simulink model "gm_kalman_ac_sim"  (R2025b)
settings: Solver=VariableStepAuto  StartTime=0.0  StopTime=StopTime  RelTol=1e-3
undefined symbols (not defined in the file or in its folder): dt, time
libraries: hdlmdlgenlib x45, hdlsllib x5, dspsrcs4 x3
settings Model: Creator=stefa  LastModifiedBy=david
settings OptimizationCC: BlockReduction=off  ConditionallyExecuteInputs=off
settings DebuggingCC: InheritedTsInSrcMsg=none

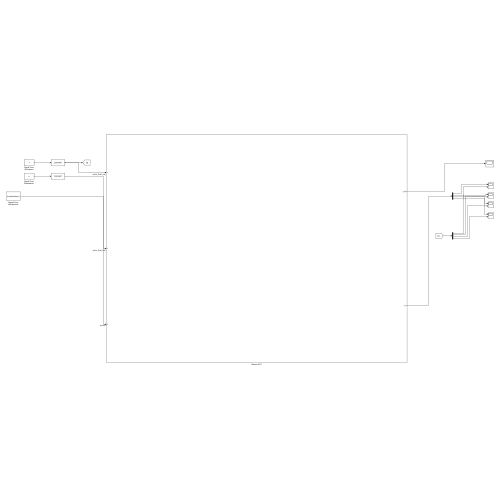
[thumbnail: Simulink's stored preview of the top-level diagram]
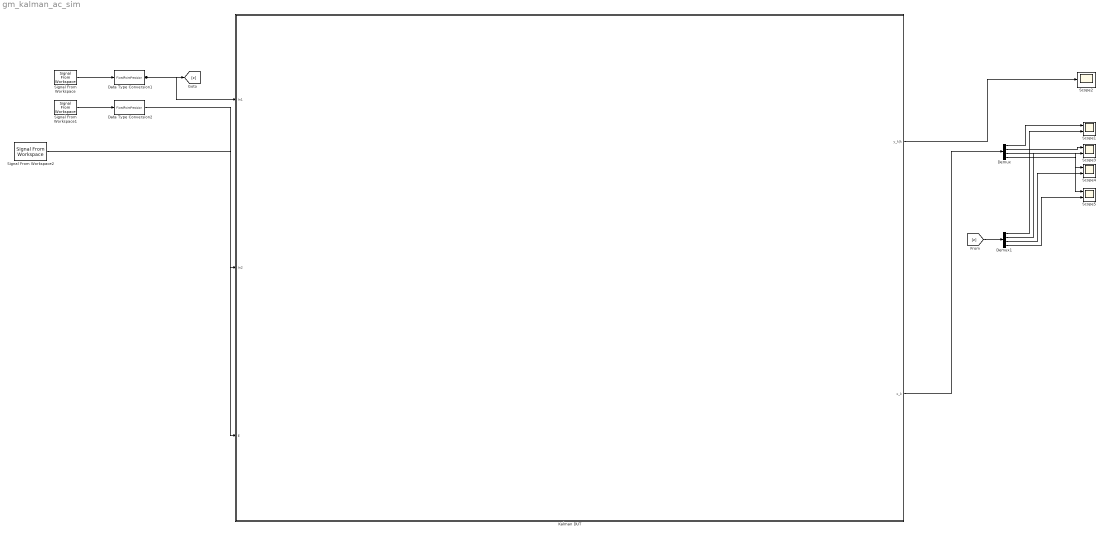
== system gm_kalman_ac_sim ==
  Data Type Conversion1 : DataTypeConversion  OutDataTypeStr=FixedPointPrecision  SaturateOnIntegerOverflow=off  RndMeth=Floor
  Data Type Conversion2 : DataTypeConversion  OutDataTypeStr=FixedPointPrecision  SaturateOnIntegerOverflow=off  RndMeth=Floor
  Demux : Demux
  Demux1 : Demux
  Kalman DUT : Subsystem
  Scope{1,3..5} (4 alike) : Scope  NumInputPorts=2
      Scope1 settings: ActiveDisplayYMinimum=0.44600438166261591  ActiveDisplayYMaximum=2.0535397271105578  DataLoggingSaveFormat=Array
      Scope3 settings: ActiveDisplayYMinimum=-1  ActiveDisplayYMaximum=1  DataLoggingVariableName=ScopeData2  DataLoggingSaveFormat=Array
      Scope4 settings: ActiveDisplayYMinimum=-2.08087494415443  ActiveDisplayYMaximum=12.219950065546442  DataLoggingVariableName=ScopeData3  DataLoggingSaveFormat=Array
      Scope5 settings: ActiveDisplayYMinimum=-0.36244737237361535  ActiveDisplayYMaximum=0.44371345235011872  DataLoggingVariableName=ScopeData4  DataLoggingSaveFormat=Array
  Scope2 : Scope
      settings: ActiveDisplayYMinimum=-0.011525178669385456  ActiveDisplayYMaximum=0.00587966952456793  DataLoggingSaveFormat=Array
  Signal From Workspace : dspsrcs4/Signal From Workspace  X=z  Ts=dt  nsamps=1  OutputAfterFinalValue=Setting to zero  ignoreOrWarnInputAndFrameLengths=off  OutputFrames=off
  Signal From Workspace1 : dspsrcs4/Signal From Workspace  X=u  Ts=dt  nsamps=1  OutputAfterFinalValue=Setting to zero  ignoreOrWarnInputAndFrameLengths=off  OutputFrames=off
  Signal From Workspace2 : dspsrcs4/Signal From Workspace  X=true(size(time))  Ts=dt  nsamps=1  OutputAfterFinalValue=Setting to zero  ignoreOrWarnInputAndFrameLengths=off  OutputFrames=off
  wires:
  Signal From Workspace2/1 -> Kalman DUT/3(E)
  Data Type Conversion2/1 -> Kalman DUT/2(In2)
  Data Type Conversion1/1 -> [z], Kalman DUT/1(In1)
  Kalman DUT/2(x_k) -> Demux/1
  Kalman DUT/1(y_k|k) -> Scope2/1
  Signal From Workspace1/1 -> Data Type Conversion2/1
  Signal From Workspace/1 -> Data Type Conversion1/1
  Demux1/4 -> Scope5/2
  Demux1/3 -> Scope4/2
  Demux1/2 -> Scope3/2
  Demux1/1 -> Scope1/2
  [z] -> Demux1/1
  Demux/4 -> Scope5/1
  Demux/3 -> Scope4/1
  Demux/2 -> Scope3/1
  Demux/1 -> Scope1/1

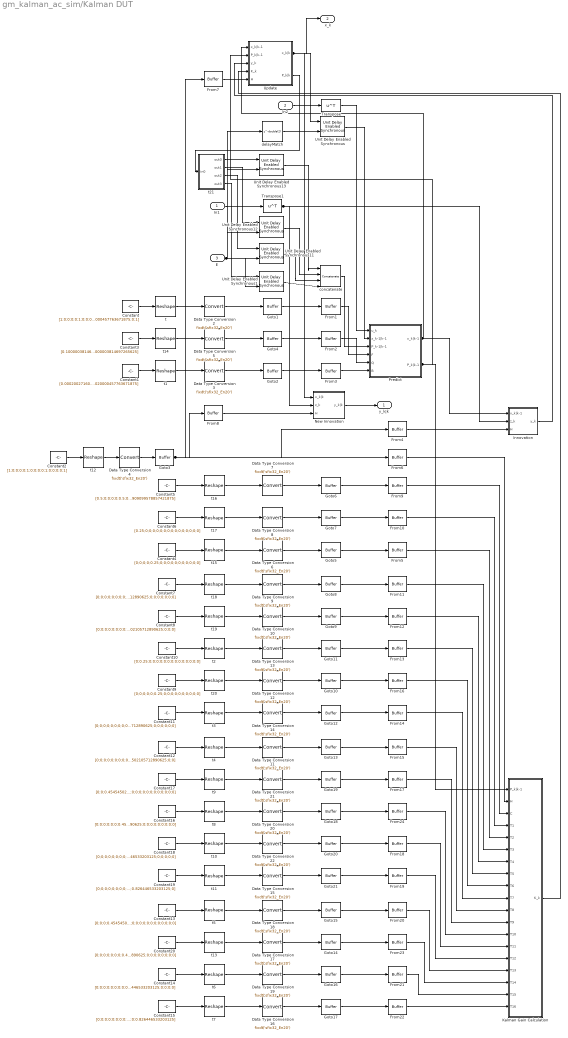
== system gm_kalman_ac_sim/Kalman DUT ==
  In1 : Inport  OutDataTypeStr=fixdt(1, 32, 20)  PortDimensions=[1 4]  SampleTime=0.02
  In2 : Inport  Port=2  OutDataTypeStr=fixdt(1, 32, 20)  PortDimensions=[1 2]  SampleTime=0.02
  E : Inport  Port=3  OutDataTypeStr=boolean  PortDimensions=1  SampleTime=0.02
  Constant : Constant  Value=[1;0;0;0;0;1;0;0;0.020000457763671875;0;1;0;0;0.020000457763671875;0;1]  OutDataTypeStr=fixdt(1, 32, 20)  SampleTime=0.02
  Constant1 : Constant  Value=[0.0002002716064453125;0;0.020000457763671875;0;0;0.0002002716064453125;0;0.020000457763671875]  OutDataTypeStr=fixdt(1, 32, 20)  SampleTime=0.02
  Constant10 : Constant  Value=[0;0.25;0;0;0;0;0;0;0;0;0;0;0;0;0;0]  OutDataTypeStr=fixdt(1, 32, 20)  SampleTime=0.02
  Constant11 : Constant  Value=[0;0;0;0;0;0;0;0;0;0.45454502105712890625;0;0;0;0;0;0]  OutDataTypeStr=fixdt(1, 32, 20)  SampleTime=0.02
  Constant12 : Constant  Value=[0;0;0;0;0;0;0;0;0;0;0;0;0;0.45454502105712890625;0;0]  OutDataTypeStr=fixdt(1, 32, 20)  SampleTime=0.02
  Constant13 : Constant  Value=[0;0;0;0.45454502105712890625;0;0;0;0;0;0;0;0;0;0;0;0]  OutDataTypeStr=fixdt(1, 32, 20)  SampleTime=0.02
  Constant14 : Constant  Value=[0;0;0;0;0;0;0;0;0;0;0;0.826446533203125;0;0;0;0]  OutDataTypeStr=fixdt(1, 32, 20)  SampleTime=0.02
  Constant15 : Constant  Value=[0;0;0;0;0;0;0;0;0;0;0;0;0;0;0;0.826446533203125]  OutDataTypeStr=fixdt(1, 32, 20)  SampleTime=0.02
  Constant16 : Constant  Value=[0;0;0;0;0;0;0.45454502105712890625;0;0;0;0;0;0;0;0;0]  OutDataTypeStr=fixdt(1, 32, 20)  SampleTime=0.02
  Constant17 : Constant  Value=[0;0;0.45454502105712890625;0;0;0;0;0;0;0;0;0;0;0;0;0]  OutDataTypeStr=fixdt(1, 32, 20)  SampleTime=0.02
  Constant18 : Constant  Value=[0;0;0;0;0;0;0;0;0;0;0.826446533203125;0;0;0;0;0]  OutDataTypeStr=fixdt(1, 32, 20)  SampleTime=0.02
  Constant19 : Constant  Value=[0;0;0;0;0;0;0;0;0;0;0;0;0;0;0.826446533203125;0]  OutDataTypeStr=fixdt(1, 32, 20)  SampleTime=0.02
  Constant2 : Constant  Value=[1;0;0;0;0;1;0;0;0;0;1;0;0;0;0;1]  OutDataTypeStr=fixdt(1, 32, 20)  SampleTime=0.02
  Constant20 : Constant  Value=[0;0;0;0;0;0;0;0.45454502105712890625;0;0;0;0;0;0;0;0]  OutDataTypeStr=fixdt(1, 32, 20)  SampleTime=0.02
  Constant3 : Constant  Value=[0.1000003814697265625;0;0;0;0;0.1000003814697265625;0;0;0;0;0.1000003814697265625;0;0;0;0;0.1000003814697265625]  OutDataTypeStr=fixdt(1, 32, 20)  SampleTime=0.02
  Constant4 : Constant  Value=[0;0;0;0;0.25;0;0;0;0;0;0;0;0;0;0;0]  OutDataTypeStr=fixdt(1, 32, 20)  SampleTime=0.02
  Constant5 : Constant  Value=[0.5;0;0;0;0;0.5;0;0;0;0;0.90909099578857421875;0;0;0;0;0.90909099578857421875]  OutDataTypeStr=fixdt(1, 32, 20)  SampleTime=0.02
  Constant6 : Constant  Value=[0.25;0;0;0;0;0;0;0;0;0;0;0;0;0;0;0]  OutDataTypeStr=fixdt(1, 32, 20)  SampleTime=0.02
  Constant7 : Constant  Value=[0;0;0;0;0;0;0;0;0.45454502105712890625;0;0;0;0;0;0;0]  OutDataTypeStr=fixdt(1, 32, 20)  SampleTime=0.02
  Constant8 : Constant  Value=[0;0;0;0;0;0;0;0;0;0;0;0;0.45454502105712890625;0;0;0]  OutDataTypeStr=fixdt(1, 32, 20)  SampleTime=0.02
  Constant9 : Constant  Value=[0;0;0;0;0;0.25;0;0;0;0;0;0;0;0;0;0]  OutDataTypeStr=fixdt(1, 32, 20)  SampleTime=0.02
  Data Type Conversion{2..22} (21 alike) : DataTypeConversion  OutDataTypeStr=fixdt('sfix32_En20')
  From{1..24} (24 alike) : hdlmdlgenlib/Buffer
  Goto{1..21} (21 alike) : hdlmdlgenlib/Buffer
  Innovation : Subsystem
  Kalman Gain Calculation : Subsystem
  New Innovation : Subsystem
  Predict : Subsystem
  Transpose : Math  Operator=transpose  SignedPower=on  OutDataTypeStr=fixdt(1, 32, 20)  RndMeth=Zero
  Transpose1 : Math  Operator=transpose  SignedPower=on  OutDataTypeStr=fixdt(1, 32, 20)  RndMeth=Zero
  Unit Delay Enabled Synchronous{,1,11..13} (5 alike) : hdlsllib/Discrete/Unit Delay Enabled Synchronous  InitialCondition=double(0)  SampleTime=-1
  Update : Subsystem
  concatenate : Concatenate  NumInputs=4  Mode=Multidimensional array  ConcatenateDimension=2
  delayMatch : Delay  DelayLength=double(2)  InitialCondition=0  SampleTime=0.02
  t{,2..20} (20 alike) : Reshape  OutputDimensionality=Customize  OutputDimensions=[4,4]
  t1 : Reshape  OutputDimensionality=Customize  OutputDimensions=[4,2]
  t21 : Subsystem
  y_k|k : Outport  SampleTime=0.02
  x_k : Outport  Port=2  SampleTime=0.02
  wires:
  t14/1 -> Data Type Conversion5/1
  From7/1 -> Update/5(H)
  Constant2/1 -> t12/1
  t21/2(out1) -> Unit Delay Enabled Synchronous12/1
  Constant1/1 -> t1/1
  t10/1 -> Data Type Conversion22/1
  Goto3/1 -> From6/1, From7/1, From8/1, From4/1
  t12/1 -> Data Type Conversion4/1
  Constant/1 -> t/1
  Constant5/1 -> t16/1
  t6/1 -> Data Type Conversion19/1
  Constant4/1 -> t15/1
  Constant6/1 -> t17/1
  Constant3/1 -> t14/1
  Data Type Conversion4/1 -> Goto3/1
  t/1 -> Data Type Conversion2/1
  delayMatch/1 -> Unit Delay Enabled Synchronous/2
  t1/1 -> Data Type Conversion3/1
  t4/1 -> Data Type Conversion11/1
  From18/1 -> Kalman Gain Calculation/14(T11)
  t2/1 -> Data Type Conversion13/1
  Constant9/1 -> t20/1
  Constant8/1 -> t19/1
  Constant7/1 -> t18/1
  Constant13/1 -> t5/1
  Constant12/1 -> t4/1
  Constant11/1 -> t3/1
  Constant10/1 -> t2/1
  Constant14/1 -> t6/1
  Constant17/1 -> t9/1
  Unit Delay Enabled Synchronous12/1 -> concatenate/2
  From16/1 -> Kalman Gain Calculation/9(T6)
  t9/1 -> Data Type Conversion21/1
  Constant20/1 -> t13/1
  Constant16/1 -> t8/1
  Constant19/1 -> t11/1
  Constant18/1 -> t10/1
  Transpose1/1 -> Innovation/2(z_k), New Innovation/2(z_k)
  Goto11/1 -> From13/1
  Constant15/1 -> t7/1
  t21/1(out0) -> Unit Delay Enabled Synchronous13/1
  t21/3(out2) -> Unit Delay Enabled Synchronous11/1
  t21/4(out3) -> Unit Delay Enabled Synchronous1/1
  In1/1 -> Transpose1/1
  E/1 -> delayMatch/1, Unit Delay Enabled Synchronous13/2, Unit Delay Enabled Synchronous11/2, Unit Delay Enabled Synchronous12/2, Unit Delay Enabled Synchronous1/2
  Data Type Conversion2/1 -> Goto1/1
  Data Type Conversion5/1 -> Goto4/1
  Data Type Conversion3/1 -> Goto2/1
  From8/1 -> New Innovation/3(H)
  t16/1 -> Data Type Conversion7/1
  t17/1 -> Data Type Conversion8/1
  t13/1 -> Data Type Conversion17/1
  t15/1 -> Data Type Conversion6/1
  Unit Delay Enabled Synchronous13/1 -> concatenate/1
  t20/1 -> Data Type Conversion12/1
  Goto8/1 -> From11/1
  t18/1 -> Data Type Conversion9/1
  t19/1 -> Data Type Conversion10/1
  t3/1 -> Data Type Conversion14/1
  t8/1 -> Data Type Conversion20/1
  t11/1 -> Data Type Conversion15/1
  Goto5/1 -> From5/1
  t7/1 -> Data Type Conversion16/1
  t5/1 -> Data Type Conversion18/1
  Update/1(x_k|k) -> Unit Delay Enabled Synchronous/1, New Innovation/1(x_k|k), x_k/1
  Update/2(P_k|k) -> t21/1(in0)
  Unit Delay Enabled Synchronous1/1 -> concatenate/4
  In2/1 -> Transpose/1
  Unit Delay Enabled Synchronous11/1 -> concatenate/3
  Predict/2(P_k|k-1) -> Update/2(P_k|k-1), Kalman Gain Calculation/1(P_k|k-1)
  Goto1/1 -> From1/1
  Goto4/1 -> From2/1
  Goto2/1 -> From3/1
  Data Type Conversion7/1 -> Goto6/1
  Data Type Conversion8/1 -> Goto7/1
  Data Type Conversion6/1 -> Goto5/1
  Data Type Conversion9/1 -> Goto8/1
  Data Type Conversion10/1 -> Goto9/1
  Data Type Conversion13/1 -> Goto11/1
  Data Type Conversion12/1 -> Goto10/1
  Data Type Conversion14/1 -> Goto12/1
  Data Type Conversion11/1 -> Goto13/1
  Data Type Conversion21/1 -> Goto19/1
  Data Type Conversion20/1 -> Goto18/1
  Data Type Conversion22/1 -> Goto20/1
  From23/1 -> Kalman Gain Calculation/17(T14)
  Unit Delay Enabled Synchronous/1 -> Predict/2(x_k-1|k-1)
  Data Type Conversion15/1 -> Goto21/1
  Data Type Conversion18/1 -> Goto15/1
  Data Type Conversion17/1 -> Goto14/1
  Data Type Conversion19/1 -> Goto16/1
  Data Type Conversion16/1 -> Goto17/1
  Transpose/1 -> Predict/1(u_k)
  concatenate/1 -> Predict/3(P_k-1|k-1)
  From1/1 -> Predict/4(F)
  From2/1 -> Predict/5(Q)
  From3/1 -> Predict/6(B)
  New Innovation/1(y_k|k) -> y_k|k/1
  Goto6/1 -> From9/1
  Goto7/1 -> From10/1
  Goto9/1 -> From12/1
  Goto10/1 -> From16/1
  Goto12/1 -> From14/1
  Goto13/1 -> From15/1
  Goto19/1 -> From17/1
  Goto18/1 -> From24/1
  Goto20/1 -> From18/1
  Goto21/1 -> From19/1
  Goto15/1 -> From20/1
  Goto14/1 -> From23/1
  Goto16/1 -> From21/1
  Goto17/1 -> From22/1
  Predict/1(x_k|k-1) -> Update/1(x_k|k-1), Innovation/1(x_k|k-1)
  From4/1 -> Innovation/3(H)
  From6/1 -> Kalman Gain Calculation/2(H)
  From9/1 -> Kalman Gain Calculation/3(C)
  From10/1 -> Kalman Gain Calculation/4(T1)
  From5/1 -> Kalman Gain Calculation/5(T2)
  From11/1 -> Kalman Gain Calculation/6(T3)
  From12/1 -> Kalman Gain Calculation/7(T4)
  From13/1 -> Kalman Gain Calculation/8(T5)
  From14/1 -> Kalman Gain Calculation/10(T7)
  From15/1 -> Kalman Gain Calculation/11(T8)
  From17/1 -> Kalman Gain Calculation/12(T9)
  From24/1 -> Kalman Gain Calculation/13(T10)
  From19/1 -> Kalman Gain Calculation/15(T12)
  From20/1 -> Kalman Gain Calculation/16(T13)
  From21/1 -> Kalman Gain Calculation/18(T15)
  From22/1 -> Kalman Gain Calculation/19(T16)
  Innovation/1(y_k) -> Update/3(y_k)
  Kalman Gain Calculation/1(K_k) -> Update/4(K_k)

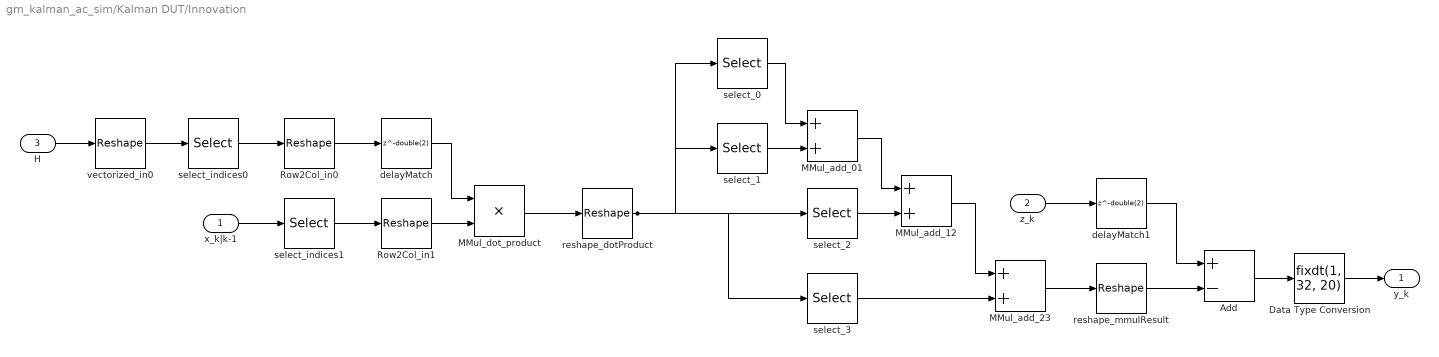
== system gm_kalman_ac_sim/Kalman DUT/Innovation ==
  x_k|k-1 : Inport  OutDataTypeStr=fixdt(1, 32, 20)  PortDimensions=[4 1]  SampleTime=0.02
  z_k : Inport  Port=2  OutDataTypeStr=fixdt(1, 32, 20)  PortDimensions=[4 1]  SampleTime=0.02
  H : Inport  Port=3  OutDataTypeStr=fixdt(1, 32, 20)  PortDimensions=[4,4]  SampleTime=0.02
  Add : Sum  Inputs=+-  OutDataTypeStr=fixdt(1, 64, 40)  AccumDataTypeStr=fixdt(1, 64, 40)  SampleTime=0.02
  Data Type Conversion : DataTypeConversion  OutDataTypeStr=fixdt(1, 32, 20)  SampleTime=0.02  SaturateOnIntegerOverflow=off  RndMeth=Floor
  MMul_add_01 : Sum  OutDataTypeStr=fixdt(1, 64, 40)  SampleTime=0.02
  MMul_add_12 : Sum  OutDataTypeStr=fixdt(1, 64, 40)  SampleTime=0.02
  MMul_add_23 : Sum  OutDataTypeStr=fixdt(1, 64, 40)  SampleTime=0.02
  MMul_dot_product : Product  Inputs=**  OutDataTypeStr=fixdt(1, 64, 40)  SampleTime=0.02
  Row2Col_in0 : Reshape  OutputDimensionality=Column vector (2-D)
  Row2Col_in1 : Reshape  OutputDimensionality=Column vector (2-D)
  delayMatch : Delay  DelayLength=double(2)  InitialCondition=0  SampleTime=0.02
  delayMatch1 : Delay  DelayLength=double(2)  InitialCondition=0  SampleTime=0.02
  reshape_dotProduct : Reshape  OutputDimensionality=Customize  OutputDimensions=[4,4]
  reshape_mmulResult : Reshape  OutputDimensionality=Customize  OutputDimensions=[4,1]
  select_0 : Selector  NumberOfDimensions=2  IndexOptions=Index vector (dialog),Select all  Indices=double(1),[]  OutputSizes=1
  select_1 : Selector  NumberOfDimensions=2  IndexOptions=Index vector (dialog),Select all  Indices=double(2),[]  OutputSizes=1
  select_2 : Selector  NumberOfDimensions=2  IndexOptions=Index vector (dialog),Select all  Indices=double(3),[]  OutputSizes=1
  select_3 : Selector  NumberOfDimensions=2  IndexOptions=Index vector (dialog),Select all  Indices=double(4),[]  OutputSizes=1
  select_indices0 : Selector  InputPortWidth=16  IndexOptions=Index vector (dialog)  Indices=double([1;5;9;13;2;6;10;14;3;7;11;15;4;8;12;16])  OutputSizes=1
  select_indices1 : Selector  InputPortWidth=4  IndexOptions=Index vector (dialog)  Indices=double([1;2;3;4;1;2;3;4;1;2;3;4;1;2;3;4])  OutputSizes=1
  vectorized_in0 : Reshape  OutputDimensionality=Row vector (2-D)
  y_k : Outport  SampleTime=0.02
  wires:
  H/1 -> vectorized_in0/1
  vectorized_in0/1 -> select_indices0/1
  select_indices0/1 -> Row2Col_in0/1
  Row2Col_in0/1 -> delayMatch/1
  MMul_add_23/1 -> reshape_mmulResult/1
  delayMatch/1 -> MMul_dot_product/1
  x_k|k-1/1 -> select_indices1/1
  Row2Col_in1/1 -> MMul_dot_product/2
  select_indices1/1 -> Row2Col_in1/1
  MMul_dot_product/1 -> reshape_dotProduct/1
  reshape_dotProduct/1 -> select_3/1, select_1/1, select_2/1, select_0/1
  select_0/1 -> MMul_add_01/1
  select_1/1 -> MMul_add_01/2
  MMul_add_01/1 -> MMul_add_12/1
  select_2/1 -> MMul_add_12/2
  select_3/1 -> MMul_add_23/2
  MMul_add_12/1 -> MMul_add_23/1
  z_k/1 -> delayMatch1/1
  delayMatch1/1 -> Add/1
  reshape_mmulResult/1 -> Add/2
  Add/1 -> Data Type Conversion/1
  Data Type Conversion/1 -> y_k/1

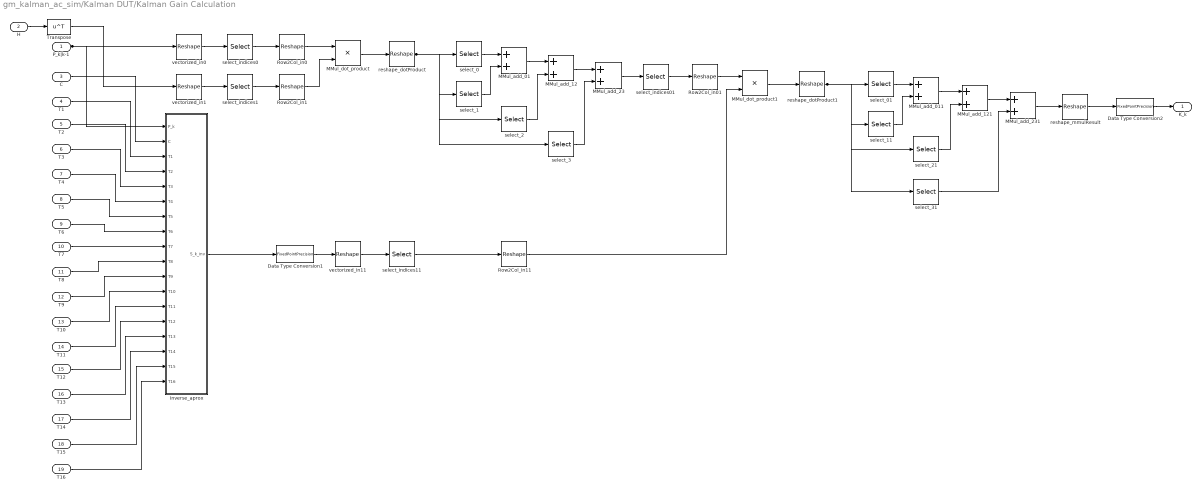
== system gm_kalman_ac_sim/Kalman DUT/Kalman Gain Calculation ==
  P_k|k-1 : Inport  OutDataTypeStr=fixdt(1, 32, 20)  PortDimensions=[4,4]  SampleTime=0.02
  H : Inport  Port=2  OutDataTypeStr=fixdt(1, 32, 20)  PortDimensions=[4,4]  SampleTime=0.02
  C : Inport  Port=3  OutDataTypeStr=fixdt(1, 32, 20)  PortDimensions=[4,4]  SampleTime=0.02
  T1 : Inport  Port=4  OutDataTypeStr=fixdt(1, 32, 20)  PortDimensions=[4,4]  SampleTime=0.02
  T2 : Inport  Port=5  OutDataTypeStr=fixdt(1, 32, 20)  PortDimensions=[4,4]  SampleTime=0.02
  T3 : Inport  Port=6  OutDataTypeStr=fixdt(1, 32, 20)  PortDimensions=[4,4]  SampleTime=0.02
  T4 : Inport  Port=7  OutDataTypeStr=fixdt(1, 32, 20)  PortDimensions=[4,4]  SampleTime=0.02
  T5 : Inport  Port=8  OutDataTypeStr=fixdt(1, 32, 20)  PortDimensions=[4,4]  SampleTime=0.02
  T6 : Inport  Port=9  OutDataTypeStr=fixdt(1, 32, 20)  PortDimensions=[4,4]  SampleTime=0.02
  T7 : Inport  Port=10  OutDataTypeStr=fixdt(1, 32, 20)  PortDimensions=[4,4]  SampleTime=0.02
  T8 : Inport  Port=11  OutDataTypeStr=fixdt(1, 32, 20)  PortDimensions=[4,4]  SampleTime=0.02
  T9 : Inport  Port=12  OutDataTypeStr=fixdt(1, 32, 20)  PortDimensions=[4,4]  SampleTime=0.02
  T10 : Inport  Port=13  OutDataTypeStr=fixdt(1, 32, 20)  PortDimensions=[4,4]  SampleTime=0.02
  T11 : Inport  Port=14  OutDataTypeStr=fixdt(1, 32, 20)  PortDimensions=[4,4]  SampleTime=0.02
  T12 : Inport  Port=15  OutDataTypeStr=fixdt(1, 32, 20)  PortDimensions=[4,4]  SampleTime=0.02
  T13 : Inport  Port=16  OutDataTypeStr=fixdt(1, 32, 20)  PortDimensions=[4,4]  SampleTime=0.02
  T14 : Inport  Port=17  OutDataTypeStr=fixdt(1, 32, 20)  PortDimensions=[4,4]  SampleTime=0.02
  T15 : Inport  Port=18  OutDataTypeStr=fixdt(1, 32, 20)  PortDimensions=[4,4]  SampleTime=0.02
  T16 : Inport  Port=19  OutDataTypeStr=fixdt(1, 32, 20)  PortDimensions=[4,4]  SampleTime=0.02
  Data Type Conversion1 : DataTypeConversion  OutDataTypeStr=FixedPointPrecision  SaturateOnIntegerOverflow=off  RndMeth=Floor
  Data Type Conversion2 : DataTypeConversion  OutDataTypeStr=FixedPointPrecision  SaturateOnIntegerOverflow=off  RndMeth=Floor
  Inverse_aprox : Subsystem
  MMul_add_01 : Sum  OutDataTypeStr=fixdt(1, 64, 40)  SampleTime=0.02
  MMul_add_011 : Sum  OutDataTypeStr=fixdt(1, 96, 60)  SampleTime=0.02
  MMul_add_12 : Sum  OutDataTypeStr=fixdt(1, 64, 40)  SampleTime=0.02
  MMul_add_121 : Sum  OutDataTypeStr=fixdt(1, 96, 60)  SampleTime=0.02
  MMul_add_23 : Sum  OutDataTypeStr=fixdt(1, 64, 40)  SampleTime=0.02
  MMul_add_231 : Sum  OutDataTypeStr=fixdt(1, 96, 60)  SampleTime=0.02
  MMul_dot_product : Product  Inputs=**  OutDataTypeStr=fixdt(1, 64, 40)  SampleTime=0.02
  MMul_dot_product1 : Product  Inputs=**  OutDataTypeStr=fixdt(1, 96, 60)  SampleTime=0.02
  Row2Col_in0 : Reshape  OutputDimensionality=Column vector (2-D)
  Row2Col_in01 : Reshape  OutputDimensionality=Column vector (2-D)
  Row2Col_in1 : Reshape  OutputDimensionality=Column vector (2-D)
  Row2Col_in11 : Reshape  OutputDimensionality=Column vector (2-D)
  Transpose : Math  Operator=transpose  SignedPower=on  OutDataTypeStr=fixdt(1, 32, 20)  RndMeth=Zero
  reshape_dotProduct : Reshape  OutputDimensionality=Customize  OutputDimensions=[4,16]
  reshape_dotProduct1 : Reshape  OutputDimensionality=Customize  OutputDimensions=[4,16]
  reshape_mmulResult : Reshape  OutputDimensionality=Customize  OutputDimensions=[4,4]
  select_0 : Selector  NumberOfDimensions=2  IndexOptions=Index vector (dialog),Select all  Indices=double(1),[]  OutputSizes=1
  select_01 : Selector  NumberOfDimensions=2  IndexOptions=Index vector (dialog),Select all  Indices=double(1),[]  OutputSizes=1
  select_1 : Selector  NumberOfDimensions=2  IndexOptions=Index vector (dialog),Select all  Indices=double(2),[]  OutputSizes=1
  select_11 : Selector  NumberOfDimensions=2  IndexOptions=Index vector (dialog),Select all  Indices=double(2),[]  OutputSizes=1
  select_2 : Selector  NumberOfDimensions=2  IndexOptions=Index vector (dialog),Select all  Indices=double(3),[]  OutputSizes=1
  select_21 : Selector  NumberOfDimensions=2  IndexOptions=Index vector (dialog),Select all  Indices=double(3),[]  OutputSizes=1
  select_3 : Selector  NumberOfDimensions=2  IndexOptions=Index vector (dialog),Select all  Indices=double(4),[]  OutputSizes=1
  select_31 : Selector  NumberOfDimensions=2  IndexOptions=Index vector (dialog),Select all  Indices=double(4),[]  OutputSizes=1
  select_indices0 : Selector  InputPortWidth=16  IndexOptions=Index vector (dialog)  Indices=double([1;5;9;13;2;6;10;14;3;7;11;15;4;8;12;16;1;5;9;13;2;6;10;14;3;7;11;15;4;8;12;16;1;5;9;13;2;6;10;14;3;7;11;15;4;8;12;16;1;5;9;13;2;6;10;14;3;7;11;15;4;8;12;16])  OutputSizes=1
  select_indices01 : Selector  InputPortWidth=16  IndexOptions=Index vector (dialog)  Indices=double([1;5;9;13;2;6;10;14;3;7;11;15;4;8;12;16;1;5;9;13;2;6;10;14;3;7;11;15;4;8;12;16;1;5;9;13;2;6;10;14;3;7;11;15;4;8;12;16;1;5;9;13;2;6;10;14;3;7;11;15;4;8;12;16])  OutputSizes=1
  select_indices1 : Selector  InputPortWidth=16  IndexOptions=Index vector (dialog)  Indices=double([1;2;3;4;1;2;3;4;1;2;3;4;1;2;3;4;5;6;7;8;5;6;7;8;5;6;7;8;5;6;7;8;9;10;11;12;9;10;11;12;9;10;11;12;9;10;11;12;13;14;15;16;13;14;15;16;13;14;15;16;13;14;15;16])  OutputSizes=1
  select_indices11 : Selector  InputPortWidth=16  IndexOptions=Index vector (dialog)  Indices=double([1;2;3;4;1;2;3;4;1;2;3;4;1;2;3;4;5;6;7;8;5;6;7;8;5;6;7;8;5;6;7;8;9;10;11;12;9;10;11;12;9;10;11;12;9;10;11;12;13;14;15;16;13;14;15;16;13;14;15;16;13;14;15;16])  OutputSizes=1
  vectorized_in0 : Reshape  OutputDimensionality=Row vector (2-D)
  vectorized_in1 : Reshape  OutputDimensionality=Row vector (2-D)
  vectorized_in11 : Reshape  OutputDimensionality=Row vector (2-D)
  K_k : Outport  SampleTime=0.02
  wires:
  C/1 -> Inverse_aprox/2(C)
  Row2Col_in1/1 -> MMul_dot_product/2
  H/1 -> Transpose/1
  Transpose/1 -> vectorized_in1/1
  P_k|k-1/1 -> Inverse_aprox/1(P_k), vectorized_in0/1
  MMul_dot_product/1 -> reshape_dotProduct/1
  T1/1 -> Inverse_aprox/3(T1)
  T3/1 -> Inverse_aprox/5(T3)
  reshape_dotProduct/1 -> select_3/1, select_2/1, select_0/1, select_1/1
  T2/1 -> Inverse_aprox/4(T2)
  select_1/1 -> MMul_add_01/2
  T6/1 -> Inverse_aprox/8(T6)
  T4/1 -> Inverse_aprox/6(T4)
  select_0/1 -> MMul_add_01/1
  T5/1 -> Inverse_aprox/7(T5)
  MMul_add_12/1 -> MMul_add_23/1
  select_2/1 -> MMul_add_12/2
  T7/1 -> Inverse_aprox/9(T7)
  MMul_add_01/1 -> MMul_add_12/1
  T8/1 -> Inverse_aprox/10(T8)
  T11/1 -> Inverse_aprox/13(T11)
  T9/1 -> Inverse_aprox/11(T9)
  MMul_add_23/1 -> select_indices01/1
  select_3/1 -> MMul_add_23/2
  T10/1 -> Inverse_aprox/12(T10)
  vectorized_in11/1 -> select_indices11/1
  T14/1 -> Inverse_aprox/16(T14)
  T12/1 -> Inverse_aprox/14(T12)
  select_indices01/1 -> Row2Col_in01/1
  select_indices11/1 -> Row2Col_in11/1
  T13/1 -> Inverse_aprox/15(T13)
  Row2Col_in11/1 -> MMul_dot_product1/2
  T15/1 -> Inverse_aprox/17(T15)
  Row2Col_in01/1 -> MMul_dot_product1/1
  T16/1 -> Inverse_aprox/18(T16)
  vectorized_in0/1 -> select_indices0/1
  vectorized_in1/1 -> select_indices1/1
  Inverse_aprox/1(S_k_inv) -> Data Type Conversion1/1
  select_indices1/1 -> Row2Col_in1/1
  select_indices0/1 -> Row2Col_in0/1
  Row2Col_in0/1 -> MMul_dot_product/1
  Data Type Conversion1/1 -> vectorized_in11/1
  select_01/1 -> MMul_add_011/1
  MMul_dot_product1/1 -> reshape_dotProduct1/1
  reshape_dotProduct1/1 -> select_31/1, select_21/1, select_11/1, select_01/1
  MMul_add_011/1 -> MMul_add_121/1
  select_11/1 -> MMul_add_011/2
  MMul_add_121/1 -> MMul_add_231/1
  select_21/1 -> MMul_add_121/2
  MMul_add_231/1 -> reshape_mmulResult/1
  select_31/1 -> MMul_add_231/2
  reshape_mmulResult/1 -> Data Type Conversion2/1
  Data Type Conversion2/1 -> K_k/1

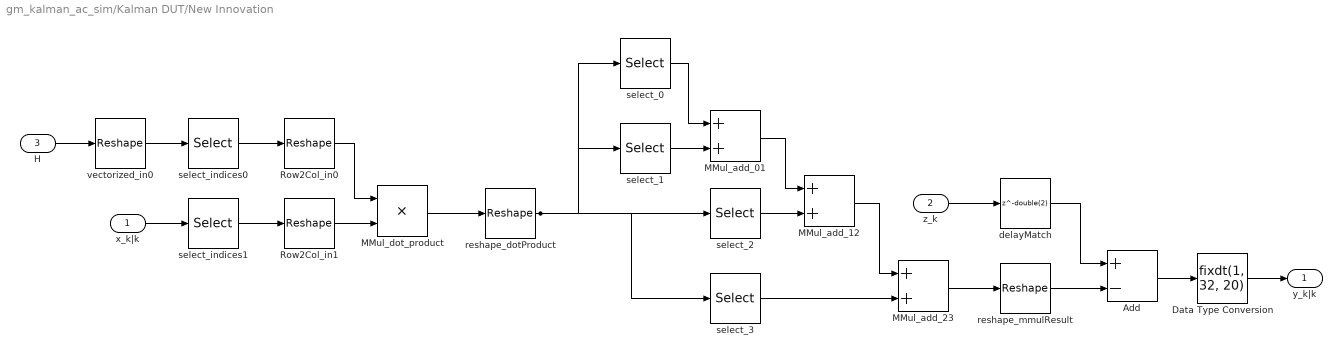
== system gm_kalman_ac_sim/Kalman DUT/New Innovation ==
  x_k|k : Inport  OutDataTypeStr=fixdt(1, 32, 20)  PortDimensions=[4 1]  SampleTime=0.02
  z_k : Inport  Port=2  OutDataTypeStr=fixdt(1, 32, 20)  PortDimensions=[4 1]  SampleTime=0.02
  H : Inport  Port=3  OutDataTypeStr=fixdt(1, 32, 20)  PortDimensions=[4,4]  SampleTime=0.02
  Add : Sum  Inputs=+-  OutDataTypeStr=fixdt(1, 64, 40)  AccumDataTypeStr=fixdt(1, 64, 40)  SampleTime=0.02
  Data Type Conversion : DataTypeConversion  OutDataTypeStr=fixdt(1, 32, 20)  SampleTime=0.02  SaturateOnIntegerOverflow=off  RndMeth=Floor
  MMul_add_01 : Sum  OutDataTypeStr=fixdt(1, 64, 40)  SampleTime=0.02
  MMul_add_12 : Sum  OutDataTypeStr=fixdt(1, 64, 40)  SampleTime=0.02
  MMul_add_23 : Sum  OutDataTypeStr=fixdt(1, 64, 40)  SampleTime=0.02
  MMul_dot_product : Product  Inputs=**  OutDataTypeStr=fixdt(1, 64, 40)  SampleTime=0.02
  Row2Col_in0 : Reshape  OutputDimensionality=Column vector (2-D)
  Row2Col_in1 : Reshape  OutputDimensionality=Column vector (2-D)
  delayMatch : Delay  DelayLength=double(2)  InitialCondition=0  SampleTime=0.02
  reshape_dotProduct : Reshape  OutputDimensionality=Customize  OutputDimensions=[4,4]
  reshape_mmulResult : Reshape  OutputDimensionality=Customize  OutputDimensions=[4,1]
  select_0 : Selector  NumberOfDimensions=2  IndexOptions=Index vector (dialog),Select all  Indices=double(1),[]  OutputSizes=1
  select_1 : Selector  NumberOfDimensions=2  IndexOptions=Index vector (dialog),Select all  Indices=double(2),[]  OutputSizes=1
  select_2 : Selector  NumberOfDimensions=2  IndexOptions=Index vector (dialog),Select all  Indices=double(3),[]  OutputSizes=1
  select_3 : Selector  NumberOfDimensions=2  IndexOptions=Index vector (dialog),Select all  Indices=double(4),[]  OutputSizes=1
  select_indices0 : Selector  InputPortWidth=16  IndexOptions=Index vector (dialog)  Indices=double([1;5;9;13;2;6;10;14;3;7;11;15;4;8;12;16])  OutputSizes=1
  select_indices1 : Selector  InputPortWidth=4  IndexOptions=Index vector (dialog)  Indices=double([1;2;3;4;1;2;3;4;1;2;3;4;1;2;3;4])  OutputSizes=1
  vectorized_in0 : Reshape  OutputDimensionality=Row vector (2-D)
  y_k|k : Outport  SampleTime=0.02
  wires:
  H/1 -> vectorized_in0/1
  vectorized_in0/1 -> select_indices0/1
  select_indices1/1 -> Row2Col_in1/1
  select_indices0/1 -> Row2Col_in0/1
  x_k|k/1 -> select_indices1/1
  Row2Col_in1/1 -> MMul_dot_product/2
  Row2Col_in0/1 -> MMul_dot_product/1
  select_0/1 -> MMul_add_01/1
  MMul_dot_product/1 -> reshape_dotProduct/1
  reshape_dotProduct/1 -> select_3/1, select_2/1, select_1/1, select_0/1
  MMul_add_01/1 -> MMul_add_12/1
  select_1/1 -> MMul_add_01/2
  MMul_add_12/1 -> MMul_add_23/1
  select_2/1 -> MMul_add_12/2
  MMul_add_23/1 -> reshape_mmulResult/1
  select_3/1 -> MMul_add_23/2
  z_k/1 -> delayMatch/1
  delayMatch/1 -> Add/1
  reshape_mmulResult/1 -> Add/2
  Add/1 -> Data Type Conversion/1
  Data Type Conversion/1 -> y_k|k/1

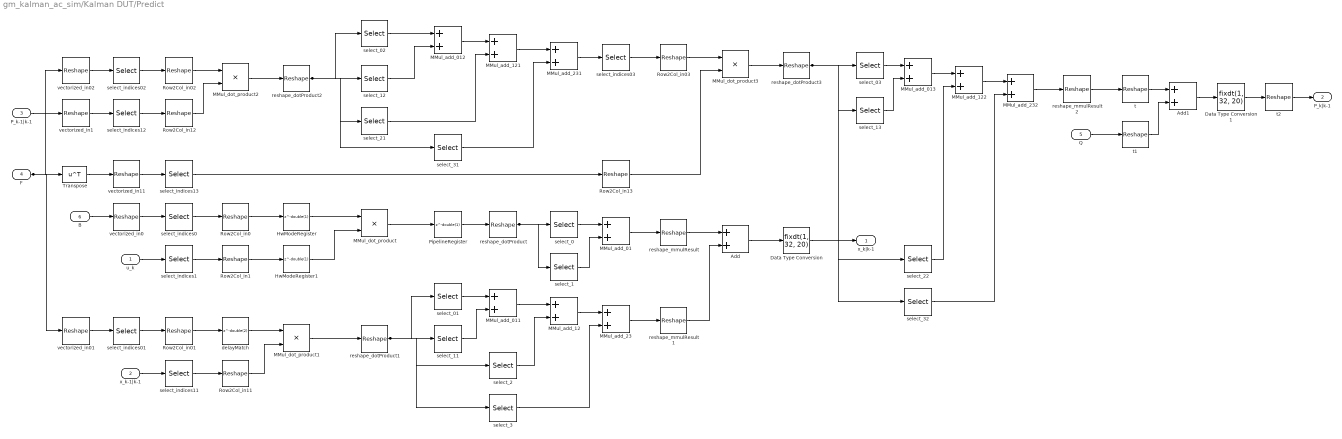
== system gm_kalman_ac_sim/Kalman DUT/Predict ==
  u_k : Inport  OutDataTypeStr=fixdt(1, 32, 20)  PortDimensions=[2 1]  SampleTime=0.02
  x_k-1|k-1 : Inport  Port=2  OutDataTypeStr=fixdt(1, 32, 20)  PortDimensions=[4 1]  SampleTime=0.02
  P_k-1|k-1 : Inport  Port=3  OutDataTypeStr=fixdt(1, 32, 20)  PortDimensions=[4,4]  SampleTime=0.02
  F : Inport  Port=4  OutDataTypeStr=fixdt(1, 32, 20)  PortDimensions=[4,4]  SampleTime=0.02
  Q : Inport  Port=5  OutDataTypeStr=fixdt(1, 32, 20)  PortDimensions=[4,4]  SampleTime=0.02
  B : Inport  Port=6  OutDataTypeStr=fixdt(1, 32, 20)  PortDimensions=[4,2]  SampleTime=0.02
  Add : Sum  OutDataTypeStr=fixdt(1, 64, 40)  AccumDataTypeStr=fixdt(1, 64, 40)  SampleTime=0.02
  Add1 : Sum  OutDataTypeStr=fixdt(1, 96, 60)  AccumDataTypeStr=fixdt(1, 96, 60)  SampleTime=0.02
  Data Type Conversion : DataTypeConversion  OutDataTypeStr=fixdt(1, 32, 20)  SampleTime=0.02  SaturateOnIntegerOverflow=off  RndMeth=Floor
  Data Type Conversion1 : DataTypeConversion  OutDataTypeStr=fixdt(1, 32, 20)  SampleTime=0.02  SaturateOnIntegerOverflow=off  RndMeth=Floor
  HwModeRegister : Delay  DelayLength=double(1)  InitialCondition=0  SampleTime=0.02
  HwModeRegister1 : Delay  DelayLength=double(1)  InitialCondition=0  SampleTime=0.02
  MMul_add_01 : Sum  OutDataTypeStr=fixdt(1, 64, 40)  SampleTime=0.02
  MMul_add_011 : Sum  OutDataTypeStr=fixdt(1, 64, 40)  SampleTime=0.02
  MMul_add_012 : Sum  OutDataTypeStr=fixdt(1, 64, 40)  SampleTime=0.02
  MMul_add_013 : Sum  OutDataTypeStr=fixdt(1, 96, 60)  SampleTime=0.02
  MMul_add_{12,23,121,231} (4 alike) : Sum  OutDataTypeStr=fixdt(1, 64, 40)  SampleTime=0.02
  MMul_add_122 : Sum  OutDataTypeStr=fixdt(1, 96, 60)  SampleTime=0.02
  MMul_add_232 : Sum  OutDataTypeStr=fixdt(1, 96, 60)  SampleTime=0.02
  MMul_dot_product : Product  Inputs=**  OutDataTypeStr=fixdt(1, 64, 40)  SampleTime=0.02
  MMul_dot_product1 : Product  Inputs=**  OutDataTypeStr=fixdt(1, 64, 40)  SampleTime=0.02
  MMul_dot_product2 : Product  Inputs=**  OutDataTypeStr=fixdt(1, 64, 40)  SampleTime=0.02
  MMul_dot_product3 : Product  Inputs=**  OutDataTypeStr=fixdt(1, 96, 60)  SampleTime=0.02
  PipelineRegister : Delay  DelayLength=double(1)  InitialCondition=0  SampleTime=0.02
  Row2Col_in{0..1,11..13} (5 alike) : Reshape  OutputDimensionality=Column vector (2-D)
  Row2Col_in01 : Reshape  OutputDimensionality=Column vector (2-D)
  Row2Col_in02 : Reshape  OutputDimensionality=Column vector (2-D)
  Row2Col_in03 : Reshape  OutputDimensionality=Column vector (2-D)
  Transpose : Math  Operator=transpose  SignedPower=on  OutDataTypeStr=fixdt(1, 32, 20)  RndMeth=Zero
  delayMatch : Delay  DelayLength=double(2)  InitialCondition=0  SampleTime=0.02
  reshape_dotProduct : Reshape  OutputDimensionality=Customize  OutputDimensions=[2,4]
  reshape_dotProduct1 : Reshape  OutputDimensionality=Customize  OutputDimensions=[4,4]
  reshape_dotProduct2 : Reshape  OutputDimensionality=Customize  OutputDimensions=[4,16]
  reshape_dotProduct3 : Reshape  OutputDimensionality=Customize  OutputDimensions=[4,16]
  reshape_mmulResult : Reshape  OutputDimensionality=Customize  OutputDimensions=[4,1]
  reshape_mmulResult1 : Reshape  OutputDimensionality=Customize  OutputDimensions=[4,1]
  reshape_mmulResult2 : Reshape  OutputDimensionality=Customize  OutputDimensions=[4,4]
  select_0 : Selector  NumberOfDimensions=2  IndexOptions=Index vector (dialog),Select all  Indices=double(1),[]  OutputSizes=1
  select_01 : Selector  NumberOfDimensions=2  IndexOptions=Index vector (dialog),Select all  Indices=double(1),[]  OutputSizes=1
  select_02 : Selector  NumberOfDimensions=2  IndexOptions=Index vector (dialog),Select all  Indices=double(1),[]  OutputSizes=1
  select_03 : Selector  NumberOfDimensions=2  IndexOptions=Index vector (dialog),Select all  Indices=double(1),[]  OutputSizes=1
  select_{1,11..13} (4 alike) : Selector  NumberOfDimensions=2  IndexOptions=Index vector (dialog),Select all  Indices=double(2),[]  OutputSizes=1
  select_2 : Selector  NumberOfDimensions=2  IndexOptions=Index vector (dialog),Select all  Indices=double(3),[]  OutputSizes=1
  select_21 : Selector  NumberOfDimensions=2  IndexOptions=Index vector (dialog),Select all  Indices=double(3),[]  OutputSizes=1
  select_22 : Selector  NumberOfDimensions=2  IndexOptions=Index vector (dialog),Select all  Indices=double(3),[]  OutputSizes=1
  select_3 : Selector  NumberOfDimensions=2  IndexOptions=Index vector (dialog),Select all  Indices=double(4),[]  OutputSizes=1
  select_31 : Selector  NumberOfDimensions=2  IndexOptions=Index vector (dialog),Select all  Indices=double(4),[]  OutputSizes=1
  select_32 : Selector  NumberOfDimensions=2  IndexOptions=Index vector (dialog),Select all  Indices=double(4),[]  OutputSizes=1
  select_indices0 : Selector  InputPortWidth=8  IndexOptions=Index vector (dialog)  Indices=double([1;5;2;6;3;7;4;8])  OutputSizes=1
  select_indices01 : Selector  InputPortWidth=16  IndexOptions=Index vector (dialog)  Indices=double([1;5;9;13;2;6;10;14;3;7;11;15;4;8;12;16])  OutputSizes=1
  select_indices02 : Selector  InputPortWidth=16  IndexOptions=Index vector (dialog)  Indices=double([1;5;9;13;2;6;10;14;3;7;11;15;4;8;12;16;1;5;9;13;2;6;10;14;3;7;11;15;4;8;12;16;1;5;9;13;2;6;10;14;3;7;11;15;4;8;12;16;1;5;9;13;2;6;10;14;3;7;11;15;4;8;12;16])  OutputSizes=1
  select_indices03 : Selector  InputPortWidth=16  IndexOptions=Index vector (dialog)  Indices=double([1;5;9;13;2;6;10;14;3;7;11;15;4;8;12;16;1;5;9;13;2;6;10;14;3;7;11;15;4;8;12;16;1;5;9;13;2;6;10;14;3;7;11;15;4;8;12;16;1;5;9;13;2;6;10;14;3;7;11;15;4;8;12;16])  OutputSizes=1
  select_indices1 : Selector  InputPortWidth=2  IndexOptions=Index vector (dialog)  Indices=double([1;2;1;2;1;2;1;2])  OutputSizes=1
  select_indices11 : Selector  InputPortWidth=4  IndexOptions=Index vector (dialog)  Indices=double([1;2;3;4;1;2;3;4;1;2;3;4;1;2;3;4])  OutputSizes=1
  select_indices12 : Selector  InputPortWidth=16  IndexOptions=Index vector (dialog)  Indices=double([1;2;3;4;1;2;3;4;1;2;3;4;1;2;3;4;5;6;7;8;5;6;7;8;5;6;7;8;5;6;7;8;9;10;11;12;9;10;11;12;9;10;11;12;9;10;11;12;13;14;15;16;13;14;15;16;13;14;15;16;13;14;15;16])  OutputSizes=1
  select_indices13 : Selector  InputPortWidth=16  IndexOptions=Index vector (dialog)  Indices=double([1;2;3;4;1;2;3;4;1;2;3;4;1;2;3;4;5;6;7;8;5;6;7;8;5;6;7;8;5;6;7;8;9;10;11;12;9;10;11;12;9;10;11;12;9;10;11;12;13;14;15;16;13;14;15;16;13;14;15;16;13;14;15;16])  OutputSizes=1
  t : Reshape  OutputDimensionality=Column vector (2-D)
  t1 : Reshape  OutputDimensionality=Column vector (2-D)
  t2 : Reshape  OutputDimensionality=Customize  OutputDimensions=[4,4]
  vectorized_in0 : Reshape  OutputDimensionality=Row vector (2-D)
  vectorized_in01 : Reshape  OutputDimensionality=Row vector (2-D)
  vectorized_in02 : Reshape  OutputDimensionality=Row vector (2-D)
  vectorized_in1 : Reshape  OutputDimensionality=Row vector (2-D)
  vectorized_in11 : Reshape  OutputDimensionality=Row vector (2-D)
  x_k|k-1 : Outport  SampleTime=0.02
  P_k|k-1 : Outport  Port=2  SampleTime=0.02
  wires:
  F/1 -> vectorized_in02/1, Transpose/1, vectorized_in01/1
  P_k-1|k-1/1 -> vectorized_in1/1
  MMul_add_23/1 -> reshape_mmulResult1/1
  vectorized_in02/1 -> select_indices02/1
  x_k-1|k-1/1 -> select_indices11/1
  select_indices02/1 -> Row2Col_in02/1
  vectorized_in1/1 -> select_indices12/1
  B/1 -> vectorized_in0/1
  Transpose/1 -> vectorized_in11/1
  MMul_add_01/1 -> reshape_mmulResult/1
  vectorized_in01/1 -> select_indices01/1
  Row2Col_in12/1 -> MMul_dot_product2/2
  select_indices12/1 -> Row2Col_in12/1
  vectorized_in11/1 -> select_indices13/1
  vectorized_in0/1 -> select_indices0/1
  u_k/1 -> select_indices1/1
  Row2Col_in01/1 -> delayMatch/1
  select_indices01/1 -> Row2Col_in01/1
  Row2Col_in02/1 -> MMul_dot_product2/1
  select_indices03/1 -> Row2Col_in03/1
  select_indices13/1 -> Row2Col_in13/1
  select_indices0/1 -> Row2Col_in0/1
  select_indices1/1 -> Row2Col_in1/1
  select_indices11/1 -> Row2Col_in11/1
  MMul_dot_product2/1 -> reshape_dotProduct2/1
  Row2Col_in0/1 -> HwModeRegister/1
  Row2Col_in1/1 -> HwModeRegister1/1
  delayMatch/1 -> MMul_dot_product1/1
  MMul_dot_product1/1 -> reshape_dotProduct1/1
  Row2Col_in11/1 -> MMul_dot_product1/2
  reshape_dotProduct2/1 -> select_21/1, select_12/1, select_02/1, select_31/1
  select_0/1 -> MMul_add_01/1
  HwModeRegister/1 -> MMul_dot_product/1
  PipelineRegister/1 -> reshape_dotProduct/1
  HwModeRegister1/1 -> MMul_dot_product/2
  select_02/1 -> MMul_add_012/1
  MMul_add_012/1 -> MMul_add_121/1
  select_12/1 -> MMul_add_012/2
  MMul_add_121/1 -> MMul_add_231/1
  select_21/1 -> MMul_add_121/2
  MMul_dot_product/1 -> PipelineRegister/1
  reshape_mmulResult/1 -> Add/1
  select_11/1 -> MMul_add_011/2
  reshape_dotProduct1/1 -> select_3/1, select_11/1, select_2/1, select_01/1
  MMul_add_231/1 -> select_indices03/1
  select_31/1 -> MMul_add_231/2
  select_01/1 -> MMul_add_011/1
  reshape_dotProduct/1 -> select_1/1, select_0/1
  MMul_add_011/1 -> MMul_add_12/1
  select_2/1 -> MMul_add_12/2
  select_3/1 -> MMul_add_23/2
  select_1/1 -> MMul_add_01/2
  MMul_add_12/1 -> MMul_add_23/1
  Row2Col_in13/1 -> MMul_dot_product3/2
  Row2Col_in03/1 -> MMul_dot_product3/1
  reshape_mmulResult1/1 -> Add/2
  select_03/1 -> MMul_add_013/1
  MMul_dot_product3/1 -> reshape_dotProduct3/1
  Add/1 -> Data Type Conversion/1
  reshape_dotProduct3/1 -> select_32/1, select_22/1, select_13/1, select_03/1
  Data Type Conversion/1 -> x_k|k-1/1
  MMul_add_013/1 -> MMul_add_122/1
  select_13/1 -> MMul_add_013/2
  select_22/1 -> MMul_add_122/2
  select_32/1 -> MMul_add_232/2
  MMul_add_122/1 -> MMul_add_232/1
  MMul_add_232/1 -> reshape_mmulResult2/1
  reshape_mmulResult2/1 -> t/1
  Q/1 -> t1/1
  t/1 -> Add1/1
  t1/1 -> Add1/2
  Add1/1 -> Data Type Conversion1/1
  Data Type Conversion1/1 -> t2/1
  t2/1 -> P_k|k-1/1

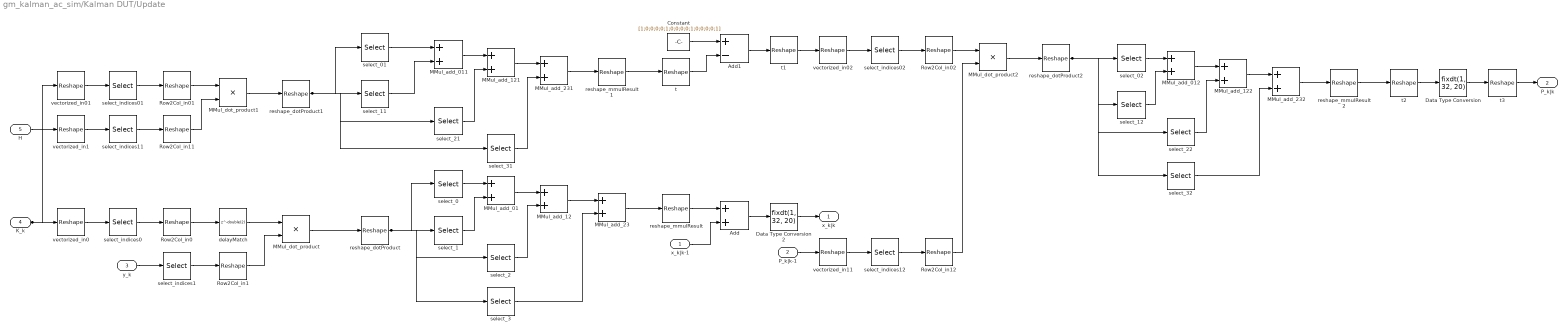
== system gm_kalman_ac_sim/Kalman DUT/Update ==
  x_k|k-1 : Inport  OutDataTypeStr=fixdt(1, 32, 20)  PortDimensions=[4 1]  SampleTime=0.02
  P_k|k-1 : Inport  Port=2  OutDataTypeStr=fixdt(1, 32, 20)  PortDimensions=[4,4]  SampleTime=0.02
  y_k : Inport  Port=3  OutDataTypeStr=fixdt(1, 32, 20)  PortDimensions=[4 1]  SampleTime=0.02
  K_k : Inport  Port=4  OutDataTypeStr=fixdt(1, 32, 20)  PortDimensions=[4,4]  SampleTime=0.02
  H : Inport  Port=5  OutDataTypeStr=fixdt(1, 32, 20)  PortDimensions=[4,4]  SampleTime=0.02
  Add : Sum  OutDataTypeStr=fixdt(1, 64, 40)  AccumDataTypeStr=fixdt(1, 64, 40)  SampleTime=0.02
  Add1 : Sum  Inputs=+-  OutDataTypeStr=fixdt(1, 64, 40)  AccumDataTypeStr=fixdt(1, 64, 40)  SampleTime=0.02
  Constant : Constant  Value=[1;0;0;0;0;1;0;0;0;0;1;0;0;0;0;1]  OutDataTypeStr=fixdt(1, 32, 20)  SampleTime=0.02
  Data Type Conversion : DataTypeConversion  OutDataTypeStr=fixdt(1, 32, 20)  SampleTime=0.02  SaturateOnIntegerOverflow=off  RndMeth=Floor
  Data Type Conversion2 : DataTypeConversion  OutDataTypeStr=fixdt(1, 32, 20)  SampleTime=0.02  SaturateOnIntegerOverflow=off  RndMeth=Floor
  MMul_add_01 : Sum  OutDataTypeStr=fixdt(1, 64, 40)  SampleTime=0.02
  MMul_add_011 : Sum  OutDataTypeStr=fixdt(1, 64, 40)  SampleTime=0.02
  MMul_add_012 : Sum  OutDataTypeStr=fixdt(1, 96, 60)  SampleTime=0.02
  MMul_add_{12,23,121,231} (4 alike) : Sum  OutDataTypeStr=fixdt(1, 64, 40)  SampleTime=0.02
  MMul_add_122 : Sum  OutDataTypeStr=fixdt(1, 96, 60)  SampleTime=0.02
  MMul_add_232 : Sum  OutDataTypeStr=fixdt(1, 96, 60)  SampleTime=0.02
  MMul_dot_product : Product  Inputs=**  OutDataTypeStr=fixdt(1, 64, 40)  SampleTime=0.02
  MMul_dot_product1 : Product  Inputs=**  OutDataTypeStr=fixdt(1, 64, 40)  SampleTime=0.02
  MMul_dot_product2 : Product  Inputs=**  OutDataTypeStr=fixdt(1, 96, 60)  SampleTime=0.02
  Row2Col_in{0..1,11..12} (4 alike) : Reshape  OutputDimensionality=Column vector (2-D)
  Row2Col_in01 : Reshape  OutputDimensionality=Column vector (2-D)
  Row2Col_in02 : Reshape  OutputDimensionality=Column vector (2-D)
  delayMatch : Delay  DelayLength=double(2)  InitialCondition=0  SampleTime=0.02
  reshape_dotProduct : Reshape  OutputDimensionality=Customize  OutputDimensions=[4,4]
  reshape_dotProduct1 : Reshape  OutputDimensionality=Customize  OutputDimensions=[4,16]
  reshape_dotProduct2 : Reshape  OutputDimensionality=Customize  OutputDimensions=[4,16]
  reshape_mmulResult : Reshape  OutputDimensionality=Customize  OutputDimensions=[4,1]
  reshape_mmulResult1 : Reshape  OutputDimensionality=Customize  OutputDimensions=[4,4]
  reshape_mmulResult2 : Reshape  OutputDimensionality=Customize  OutputDimensions=[4,4]
  select_0 : Selector  NumberOfDimensions=2  IndexOptions=Index vector (dialog),Select all  Indices=double(1),[]  OutputSizes=1
  select_01 : Selector  NumberOfDimensions=2  IndexOptions=Index vector (dialog),Select all  Indices=double(1),[]  OutputSizes=1
  select_02 : Selector  NumberOfDimensions=2  IndexOptions=Index vector (dialog),Select all  Indices=double(1),[]  OutputSizes=1
  select_1 : Selector  NumberOfDimensions=2  IndexOptions=Index vector (dialog),Select all  Indices=double(2),[]  OutputSizes=1
  select_11 : Selector  NumberOfDimensions=2  IndexOptions=Index vector (dialog),Select all  Indices=double(2),[]  OutputSizes=1
  select_12 : Selector  NumberOfDimensions=2  IndexOptions=Index vector (dialog),Select all  Indices=double(2),[]  OutputSizes=1
  select_2 : Selector  NumberOfDimensions=2  IndexOptions=Index vector (dialog),Select all  Indices=double(3),[]  OutputSizes=1
  select_21 : Selector  NumberOfDimensions=2  IndexOptions=Index vector (dialog),Select all  Indices=double(3),[]  OutputSizes=1
  select_22 : Selector  NumberOfDimensions=2  IndexOptions=Index vector (dialog),Select all  Indices=double(3),[]  OutputSizes=1
  select_3 : Selector  NumberOfDimensions=2  IndexOptions=Index vector (dialog),Select all  Indices=double(4),[]  OutputSizes=1
  select_31 : Selector  NumberOfDimensions=2  IndexOptions=Index vector (dialog),Select all  Indices=double(4),[]  OutputSizes=1
  select_32 : Selector  NumberOfDimensions=2  IndexOptions=Index vector (dialog),Select all  Indices=double(4),[]  OutputSizes=1
  select_indices0 : Selector  InputPortWidth=16  IndexOptions=Index vector (dialog)  Indices=double([1;5;9;13;2;6;10;14;3;7;11;15;4;8;12;16])  OutputSizes=1
  select_indices01 : Selector  InputPortWidth=16  IndexOptions=Index vector (dialog)  Indices=double([1;5;9;13;2;6;10;14;3;7;11;15;4;8;12;16;1;5;9;13;2;6;10;14;3;7;11;15;4;8;12;16;1;5;9;13;2;6;10;14;3;7;11;15;4;8;12;16;1;5;9;13;2;6;10;14;3;7;11;15;4;8;12;16])  OutputSizes=1
  select_indices02 : Selector  InputPortWidth=16  IndexOptions=Index vector (dialog)  Indices=double([1;5;9;13;2;6;10;14;3;7;11;15;4;8;12;16;1;5;9;13;2;6;10;14;3;7;11;15;4;8;12;16;1;5;9;13;2;6;10;14;3;7;11;15;4;8;12;16;1;5;9;13;2;6;10;14;3;7;11;15;4;8;12;16])  OutputSizes=1
  select_indices1 : Selector  InputPortWidth=4  IndexOptions=Index vector (dialog)  Indices=double([1;2;3;4;1;2;3;4;1;2;3;4;1;2;3;4])  OutputSizes=1
  select_indices11 : Selector  InputPortWidth=16  IndexOptions=Index vector (dialog)  Indices=double([1;2;3;4;1;2;3;4;1;2;3;4;1;2;3;4;5;6;7;8;5;6;7;8;5;6;7;8;5;6;7;8;9;10;11;12;9;10;11;12;9;10;11;12;9;10;11;12;13;14;15;16;13;14;15;16;13;14;15;16;13;14;15;16])  OutputSizes=1
  select_indices12 : Selector  InputPortWidth=16  IndexOptions=Index vector (dialog)  Indices=double([1;2;3;4;1;2;3;4;1;2;3;4;1;2;3;4;5;6;7;8;5;6;7;8;5;6;7;8;5;6;7;8;9;10;11;12;9;10;11;12;9;10;11;12;9;10;11;12;13;14;15;16;13;14;15;16;13;14;15;16;13;14;15;16])  OutputSizes=1
  t : Reshape  OutputDimensionality=Column vector (2-D)
  t1 : Reshape  OutputDimensionality=Customize  OutputDimensions=[4,4]
  t2 : Reshape  OutputDimensionality=Column vector (2-D)
  t3 : Reshape  OutputDimensionality=Customize  OutputDimensions=[4,4]
  vectorized_in0 : Reshape  OutputDimensionality=Row vector (2-D)
  vectorized_in01 : Reshape  OutputDimensionality=Row vector (2-D)
  vectorized_in02 : Reshape  OutputDimensionality=Row vector (2-D)
  vectorized_in1 : Reshape  OutputDimensionality=Row vector (2-D)
  vectorized_in11 : Reshape  OutputDimensionality=Row vector (2-D)
  x_k|k : Outport  SampleTime=0.02
  P_k|k : Outport  Port=2  SampleTime=0.02
  wires:
  K_k/1 -> vectorized_in01/1, vectorized_in0/1
  H/1 -> vectorized_in1/1
  MMul_add_23/1 -> reshape_mmulResult/1
  vectorized_in01/1 -> select_indices01/1
  select_indices01/1 -> Row2Col_in01/1
  select_indices11/1 -> Row2Col_in11/1
  vectorized_in1/1 -> select_indices11/1
  vectorized_in0/1 -> select_indices0/1
  Row2Col_in0/1 -> delayMatch/1
  select_indices0/1 -> Row2Col_in0/1
  y_k/1 -> select_indices1/1
  Row2Col_in01/1 -> MMul_dot_product1/1
  Row2Col_in11/1 -> MMul_dot_product1/2
  select_indices1/1 -> Row2Col_in1/1
  select_01/1 -> MMul_add_011/1
  MMul_dot_product1/1 -> reshape_dotProduct1/1
  delayMatch/1 -> MMul_dot_product/1
  MMul_dot_product/1 -> reshape_dotProduct/1
  Row2Col_in1/1 -> MMul_dot_product/2
  reshape_dotProduct1/1 -> select_31/1, select_21/1, select_11/1, select_01/1
  MMul_add_011/1 -> MMul_add_121/1
  select_11/1 -> MMul_add_011/2
  select_1/1 -> MMul_add_01/2
  reshape_dotProduct/1 -> select_3/1, select_2/1, select_1/1, select_0/1
  MMul_add_121/1 -> MMul_add_231/1
  select_21/1 -> MMul_add_121/2
  select_0/1 -> MMul_add_01/1
  MMul_add_231/1 -> reshape_mmulResult1/1
  select_31/1 -> MMul_add_231/2
  MMul_add_01/1 -> MMul_add_12/1
  select_2/1 -> MMul_add_12/2
  select_3/1 -> MMul_add_23/2
  MMul_add_12/1 -> MMul_add_23/1
  reshape_mmulResult1/1 -> t/1
  Constant/1 -> Add1/1
  MMul_add_232/1 -> reshape_mmulResult2/1
  t/1 -> Add1/2
  reshape_mmulResult/1 -> Add/1
  x_k|k-1/1 -> Add/2
  Add/1 -> Data Type Conversion2/1
  Add1/1 -> t1/1
  t3/1 -> P_k|k/1
  t1/1 -> vectorized_in02/1
  Data Type Conversion2/1 -> x_k|k/1
  P_k|k-1/1 -> vectorized_in11/1
  vectorized_in02/1 -> select_indices02/1
  Row2Col_in02/1 -> MMul_dot_product2/1
  vectorized_in11/1 -> select_indices12/1
  select_indices02/1 -> Row2Col_in02/1
  select_indices12/1 -> Row2Col_in12/1
  MMul_dot_product2/1 -> reshape_dotProduct2/1
  Row2Col_in12/1 -> MMul_dot_product2/2
  select_12/1 -> MMul_add_012/2
  reshape_dotProduct2/1 -> select_32/1, select_12/1, select_02/1, select_22/1
  select_02/1 -> MMul_add_012/1
  MMul_add_012/1 -> MMul_add_122/1
  select_22/1 -> MMul_add_122/2
  select_32/1 -> MMul_add_232/2
  MMul_add_122/1 -> MMul_add_232/1
  reshape_mmulResult2/1 -> t2/1
  t2/1 -> Data Type Conversion/1
  Data Type Conversion/1 -> t3/1

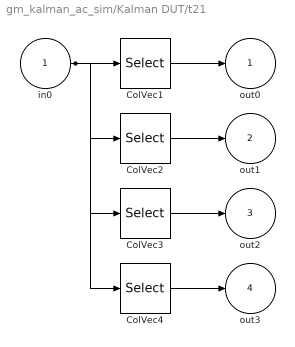
== system gm_kalman_ac_sim/Kalman DUT/t21 ==
  in0 : Inport
  ColVec1 : Selector  NumberOfDimensions=2  IndexOptions=Select all,Index vector (dialog)  Indices=1,1  OutputSizes=1,1
  ColVec2 : Selector  NumberOfDimensions=2  IndexOptions=Select all,Index vector (dialog)  Indices=1,2  OutputSizes=1,1
  ColVec3 : Selector  NumberOfDimensions=2  IndexOptions=Select all,Index vector (dialog)  Indices=1,3  OutputSizes=1,1
  ColVec4 : Selector  NumberOfDimensions=2  IndexOptions=Select all,Index vector (dialog)  Indices=1,4  OutputSizes=1,1
  out0 : Outport
  out1 : Outport  Port=2
  out2 : Outport  Port=3
  out3 : Outport  Port=4
  wires:
  in0/1 -> ColVec1/1, ColVec2/1, ColVec3/1, ColVec4/1
  ColVec1/1 -> out0/1
  ColVec2/1 -> out1/1
  ColVec3/1 -> out2/1
  ColVec4/1 -> out3/1

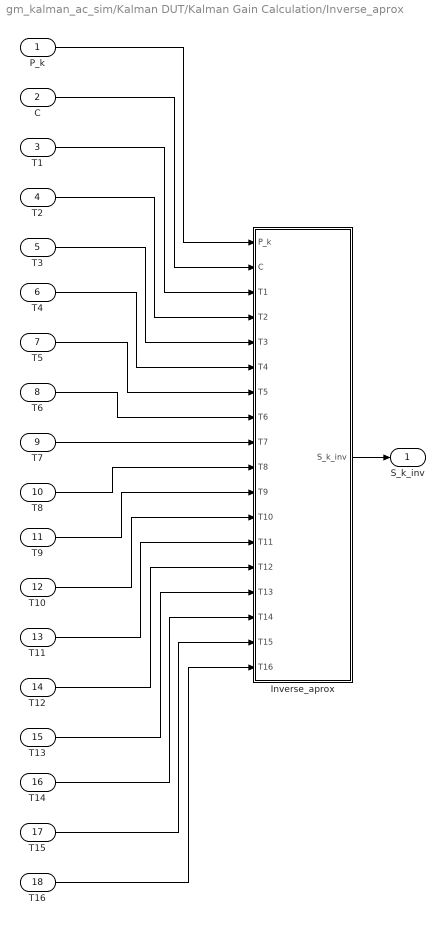
== system gm_kalman_ac_sim/Kalman DUT/Kalman Gain Calculation/Inverse_aprox ==
  P_k : Inport  OutDataTypeStr=fixdt(1, 32, 20)  PortDimensions=[4,4]  SampleTime=0.02
  C : Inport  Port=2  OutDataTypeStr=fixdt(1, 32, 20)  PortDimensions=[4,4]  SampleTime=0.02
  T1 : Inport  Port=3  OutDataTypeStr=fixdt(1, 32, 20)  PortDimensions=[4,4]  SampleTime=0.02
  T2 : Inport  Port=4  OutDataTypeStr=fixdt(1, 32, 20)  PortDimensions=[4,4]  SampleTime=0.02
  T3 : Inport  Port=5  OutDataTypeStr=fixdt(1, 32, 20)  PortDimensions=[4,4]  SampleTime=0.02
  T4 : Inport  Port=6  OutDataTypeStr=fixdt(1, 32, 20)  PortDimensions=[4,4]  SampleTime=0.02
  T5 : Inport  Port=7  OutDataTypeStr=fixdt(1, 32, 20)  PortDimensions=[4,4]  SampleTime=0.02
  T6 : Inport  Port=8  OutDataTypeStr=fixdt(1, 32, 20)  PortDimensions=[4,4]  SampleTime=0.02
  T7 : Inport  Port=9  OutDataTypeStr=fixdt(1, 32, 20)  PortDimensions=[4,4]  SampleTime=0.02
  T8 : Inport  Port=10  OutDataTypeStr=fixdt(1, 32, 20)  PortDimensions=[4,4]  SampleTime=0.02
  T9 : Inport  Port=11  OutDataTypeStr=fixdt(1, 32, 20)  PortDimensions=[4,4]  SampleTime=0.02
  T10 : Inport  Port=12  OutDataTypeStr=fixdt(1, 32, 20)  PortDimensions=[4,4]  SampleTime=0.02
  T11 : Inport  Port=13  OutDataTypeStr=fixdt(1, 32, 20)  PortDimensions=[4,4]  SampleTime=0.02
  T12 : Inport  Port=14  OutDataTypeStr=fixdt(1, 32, 20)  PortDimensions=[4,4]  SampleTime=0.02
  T13 : Inport  Port=15  OutDataTypeStr=fixdt(1, 32, 20)  PortDimensions=[4,4]  SampleTime=0.02
  T14 : Inport  Port=16  OutDataTypeStr=fixdt(1, 32, 20)  PortDimensions=[4,4]  SampleTime=0.02
  T15 : Inport  Port=17  OutDataTypeStr=fixdt(1, 32, 20)  PortDimensions=[4,4]  SampleTime=0.02
  T16 : Inport  Port=18  OutDataTypeStr=fixdt(1, 32, 20)  PortDimensions=[4,4]  SampleTime=0.02
  Inverse_aprox : MATLAB Function  TreatAsAtomicUnit=on
  S_k_inv : Outport  SampleTime=0.02
  wires:
  C/1 -> Inverse_aprox/2(C)
  P_k/1 -> Inverse_aprox/1(P_k)
  T2/1 -> Inverse_aprox/4(T2)
  T1/1 -> Inverse_aprox/3(T1)
  T3/1 -> Inverse_aprox/5(T3)
  T5/1 -> Inverse_aprox/7(T5)
  T4/1 -> Inverse_aprox/6(T4)
  T8/1 -> Inverse_aprox/10(T8)
  T6/1 -> Inverse_aprox/8(T6)
  T7/1 -> Inverse_aprox/9(T7)
  T9/1 -> Inverse_aprox/11(T9)
  T10/1 -> Inverse_aprox/12(T10)
  T13/1 -> Inverse_aprox/15(T13)
  T11/1 -> Inverse_aprox/13(T11)
  T12/1 -> Inverse_aprox/14(T12)
  T16/1 -> Inverse_aprox/18(T16)
  T14/1 -> Inverse_aprox/16(T14)
  T15/1 -> Inverse_aprox/17(T15)
  Inverse_aprox/1(S_k_inv) -> S_k_inv/1

== matlab function gm_kalman_ac_sim/Kalman DUT/Kalman Gain Calculation/Inverse_aprox/Inverse_aprox ==
  data: S_k_inv output; P_k input; C input; T1 input; T2 input; T3 input; T4 input; T5 input; T6 input; T7 input; T8 input; T9 input; T10 input; T11 input; T12 input; T13 input; T14 input; T15 input; T16 input
function S_k_inv = inverse_aprox(P_k, C, T1, T2, T3, T4, T5, T6, T7, T8, T9, T10, T11, T12, T13, T14, T15, T16)
    Z = P_k - fi(eye(4),true, 66, 40);
    sum = fi(zeros(4,4),true, 66, 40);
    sum = sum + T1*Z(1,1);
    sum = sum + T2*Z(1,2);
    sum = sum + T3*Z(1,3);
    sum = sum + T4*Z(1,4);
    sum = sum + T5*Z(2,1);
    sum = sum + T6*Z(2,2);
    sum = sum + T7*Z(2,3);
    sum = sum + T8*Z(2,4);
    sum = sum + T9*Z(3,1);
    sum = sum + T10*Z(3,2);
    sum = sum + T11*Z(3,3);
    sum = sum + T12*Z(3,4);
    sum = sum + T13*Z(4,1);
    sum = sum + T14*Z(4,2);
    sum = sum + T15*Z(4,3);
    sum = sum + T16*Z(4,4);    
    S_k_inv = C - fi(sum, true, 32, 20);
end
